simulink model "Convex_MPC_Cheetah"  (R2020b)
settings: Solver=VariableStepAuto  StartTime=0.0  StopTime=3  RelTol=1e-3
values from neighbouring files (symbols this model uses):
  fp_0 = fp_example    [Main.m]
  px_dot_desired = 1    [Main.m]
  py_dot_desired = 0    [Main.m]
  pz_desired = h_body    (= 0.2)    [Main.m]
  RPY0 = [0; 0; 0]    [Main.m]
  Xs0 = [p0; dp0; omega0; R0(:)]    [Main.m]
  yaw_dot_desired = 0    [Main.m]
undefined symbols (not defined in the file or in its folder): convexMPC, derivedEulerangles, F_example, fp_example, genTrajectory, robotDynamics
settings Model: Creator=Administrator  LastModifiedBy=Administrator

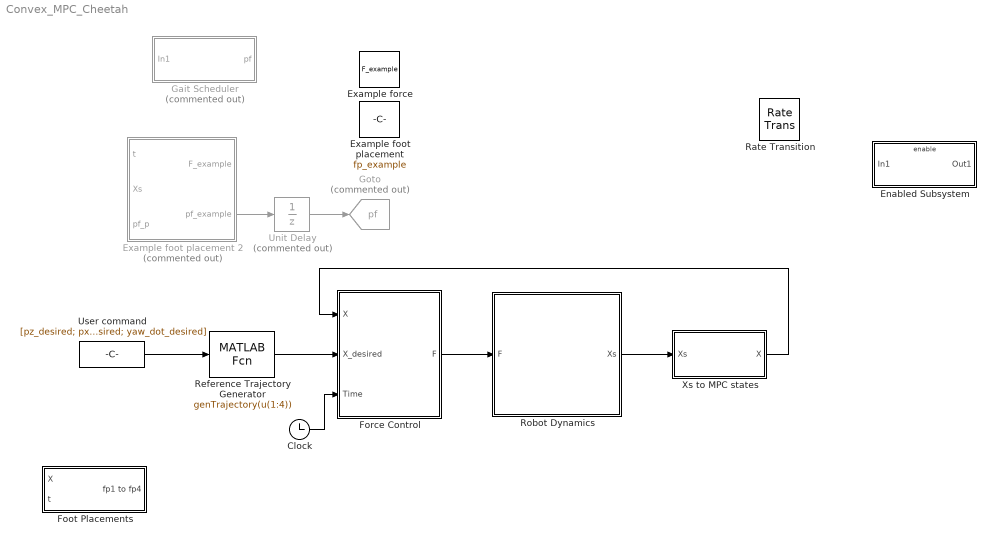
== system Convex_MPC_Cheetah ==
  Clock : Clock
  Enabled Subsystem : Subsystem  TreatAsAtomicUnit=on
  Example foot placement : Constant  Value=fp_example
  Example foot placement 2 : MATLAB Function  Commented=on  TreatAsAtomicUnit=on
  Example force : Constant  Value=F_example
  Foot Placements : Subsystem
  Force Control : Subsystem
  Gait Scheduler : Subsystem  Commented=on
  Goto : Goto  Commented=on  GotoTag=pf  TagVisibility=global
  Rate Transition : RateTransition
  Reference Trajectory Generator : MATLABFcn  MATLABFcn=genTrajectory(u(1:4))
  Robot Dynamics : Subsystem
  Unit Delay : UnitDelay  Commented=on  InitialCondition=fp_0  SampleTime=-1  HasFrameUpgradeWarning=on
  User command : Constant  Value=[pz_desired; px_dot_desired; py_dot_desired; yaw_dot_desired]
  Xs to MPC states : Subsystem
  wires:
  Robot Dynamics/1(Xs) -> Xs to MPC states/1(Xs)
  Example foot placement 2/2(pf_example) -> Unit Delay/1
  Unit Delay/1 -> Goto/1
  Force Control/1(F) -> Robot Dynamics/1(F)
  Xs to MPC states/1(X) -> Force Control/1(X)
  Reference Trajectory Generator/1 -> Force Control/2(X_desired)
  User command/1 -> Reference Trajectory Generator/1
  Clock/1 -> Force Control/3(Time)

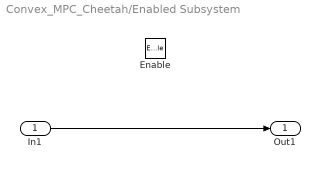
== system Convex_MPC_Cheetah/Enabled Subsystem ==
  In1 : Inport
  Enable : EnablePort
  Out1 : Outport
  wires:
  In1/1 -> Out1/1

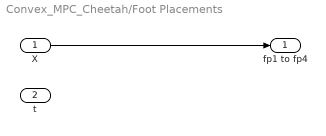
== system Convex_MPC_Cheetah/Foot Placements ==
  X : Inport
  t : Inport  Port=2
  fp1 to fp4 : Outport
  wires:
  X/1 -> fp1 to fp4/1

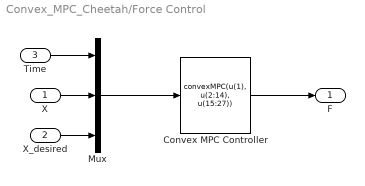
== system Convex_MPC_Cheetah/Force Control ==
  X : Inport
  X_desired : Inport  Port=2
  Time : Inport  Port=3
  Convex MPC Controller : MATLABFcn  MATLABFcn=convexMPC(u(1), u(2:14), u(15:27))
  Mux : Mux  Inputs=3
  F : Outport
  wires:
  X_desired/1 -> Mux/3
  X/1 -> Mux/2
  Time/1 -> Mux/1
  Mux/1 -> Convex MPC Controller/1
  Convex MPC Controller/1 -> F/1

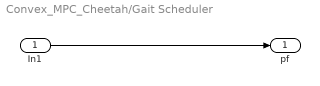
== system Convex_MPC_Cheetah/Gait Scheduler ==
  In1 : Inport
  pf : Outport
  wires:
  In1/1 -> pf/1

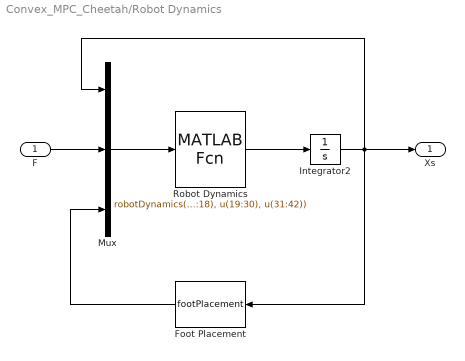
== system Convex_MPC_Cheetah/Robot Dynamics ==
  F : Inport
  Foot Placement : MATLABFcn  MATLABFcn=footPlacement  OutputDimensions=[18 1]  OutputSignalType=real  Output1D=off
  Integrator2 : Integrator  InitialCondition=Xs0
  Mux : Mux  Inputs=3
  Robot Dynamics : MATLABFcn  MATLABFcn=robotDynamics(u(1:18), u(19:30), u(31:42))  OutputDimensions=[18 1]  OutputSignalType=real  Output1D=off
  Xs : Outport
  wires:
  Foot Placement/1 -> Mux/3
  Mux/1 -> Robot Dynamics/1
  Robot Dynamics/1 -> Integrator2/1
  Integrator2/1 -> Foot Placement/1, Xs/1, Mux/1
  F/1 -> Mux/2

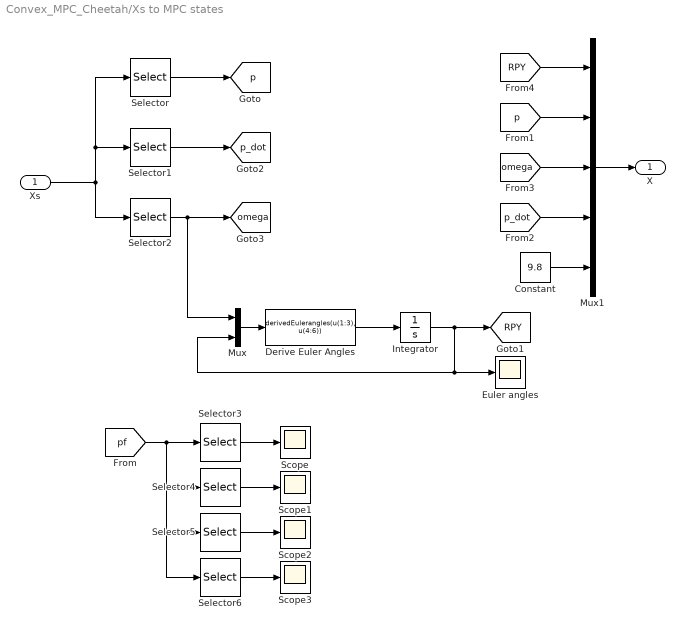
== system Convex_MPC_Cheetah/Xs to MPC states ==
  Xs : Inport
  Constant : Constant  Value=9.8
  Derive Euler Angles : MATLABFcn  MATLABFcn=derivedEulerangles(u(1:3), u(4:6))  OutputDimensions=[3 1]  OutputSignalType=real  Output1D=off
  Euler angles : Scope
  Integrator : Integrator  InitialCondition=RPY0
  Mux : Mux  Inputs=2
  Mux1 : Mux  Inputs=5
  Scope{,1..3} (4 alike) : Scope
  Selector : Selector  InputPortWidth=18  IndexOptions=Index vector (dialog)  Indices=[1:3]  OutputSizes=1
  Selector1 : Selector  InputPortWidth=18  IndexOptions=Index vector (dialog)  Indices=[4:6]  OutputSizes=1
  Selector2 : Selector  InputPortWidth=18  IndexOptions=Index vector (dialog)  Indices=[7:9]  OutputSizes=1
  Selector3 : Selector  InputPortWidth=12  IndexOptions=Index vector (dialog)  Indices=[1:3]  OutputSizes=1
  Selector4 : Selector  InputPortWidth=12  IndexOptions=Index vector (dialog)  Indices=[4:6]  OutputSizes=1
  Selector5 : Selector  InputPortWidth=12  IndexOptions=Index vector (dialog)  Indices=[7:9]  OutputSizes=1
  Selector6 : Selector  InputPortWidth=12  IndexOptions=Index vector (dialog)  Indices=[10:12]  OutputSizes=1
  X : Outport
  tag scope: RPY=global, omega=global, p=global, p_dot=global
  wires:
  Xs/1 -> Selector/1, Selector1/1, Selector2/1
  Selector2/1 -> [omega], Mux/1
  Selector1/1 -> [p_dot]
  Selector/1 -> [p]
  Mux/1 -> Derive Euler Angles/1
  Derive Euler Angles/1 -> Integrator/1
  Integrator/1 -> Euler angles/1, Mux/2, [RPY]
  [pf] -> Selector4/1, Selector5/1, Selector6/1, Selector3/1
  Selector3/1 -> Scope/1
  Selector6/1 -> Scope3/1
  Selector5/1 -> Scope2/1
  Selector4/1 -> Scope1/1
  Mux1/1 -> X/1
  [RPY] -> Mux1/1
  [p] -> Mux1/2
  [omega] -> Mux1/3
  [p_dot] -> Mux1/4
  Constant/1 -> Mux1/5

== matlab function Convex_MPC_Cheetah/Example foot placement 2 ==
  data: t input; F_example output; pf_example output; Xs input; pf_p input
function [F_example, pf_example] = fcn(t, Xs, pf_p)
% Trotting gait example

p = Xs(1:3); p_dot = Xs(4:6);
pf_p = reshape(pf_p, [3, 4]);

l_body = 0.6;
w_body = 0.256;
h_body = 0.2;

T_gait = 0.5;
T_stance = T_gait/2;

if mod(floor(t/T_gait), 2) == 0
    % foot 1 and 3 are in contact
    F_example = [[43*0.6/2; 0; 43*9.8/2]; [0; 0; 0]; ...
                 [-43*0.6/4; 0; 43*9.8/2]; [0; 0; 0]];
    pf1 = pf_p(:, 1);
    pf2 = p + p_dot*T_stance/2 + [-w_body/2;  l_body/2; -h_body];
    pf3 = pf_p(:, 3);
    pf4 = p + p_dot*T_stance/2 + [ w_body/2; -l_body/2; -h_body];
    pf_example = [pf1; pf2; pf3; pf4];
%     pf_example = [[-w_body/2; -l_body/2; -h_body]; ...
%                   [-w_body/2;  l_body/2; -h_body]; ...
%                   [ w_body/2;  l_body/2; -h_body]; ...
%                   [ w_body/2; -l_body/2; -h_body]];
else
    % foot 2 and 4 are in contact
    F_example = [[0; 0; 0]; [43*0.6/2; 0; 43*9.8/2]; ...
                 [0; 0; 0]; [-43*0.6/4; 0; 43*9.8/2]];
    pf1 = p + p_dot*T_stance/2 + [-w_body/2; -l_body/2; -h_body];
    pf2 = pf_p(:, 2);
    pf3 = p + p_dot*T_stance/2 + [ w_body/2;  l_body/2; -h_body];
    pf4 = pf_p(:, 4);
    pf_example = [pf1; pf2; pf3; pf4];
%     pf_example = [[-w_body/2; -l_body/2; -h_body]; ...
%                   [-w_body/2;  l_body/2; -h_body]; ...
%                   [ w_body/2;  l_body/2; -h_body]; ...
%                   [ w_body/2; -l_body/2; -h_body]];
end

end
